simulink library "MCI_lib"  (Simulink 7.5)
settings: Solver=ode45  StartTime=0.0  StopTime=10.0  RelTol=1e-3
values from neighbouring files (symbols this model uses):
  pMCI_bool_MotCtrlTqLimEna_C = Simulink.Parameter    [MCI_par.m]
  pMCI_m_TireDiam_C = Simulink.Parameter    [MCI_par.m]
  pMCI_Nm_DrvTqLim_C = Simulink.Parameter    [MCI_par.m]
  pMCI_Nm_RcpTqLim_C = Simulink.Parameter    [MCI_par.m]
  pMCI_ratio_DrvEff_MAP = Simulink.Parameter    [MCI_par.m]
  pMCI_ratio_KmPerHrToMtrPerSec_C = Simulink.Parameter    [MCI_par.m]
  pMCI_ratio_TrsmRat_C = Simulink.Parameter    [MCI_par.m]
  pMCI_rpm_InsteadVld_C = Simulink.Parameter    [MCI_par.m]
  pMCI_s_NoOfSec_C = Simulink.Parameter    [MCI_par.m]
undefined symbols (not defined in the file or in its folder): MotCtrlWrkStsTyp, p_bool_False_M, p_bool_True_M, p_st_DrvModeFlg_C
libraries: BaseOperationLib_Browser x79, PES_CZ_FAW x6, simulink x1
(part 2 of 2)

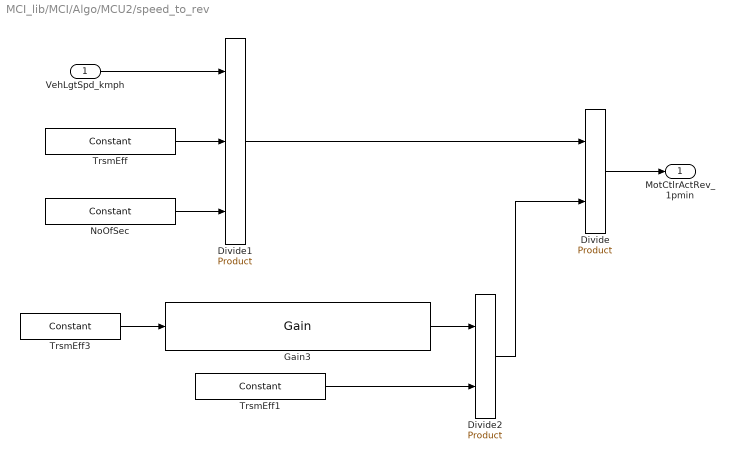
== system MCI_lib/MCI/Algo/MCU2/speed_to_rev ==
  VehLgtSpd_kmph : Inport
  Divide : BaseOperationLib_Browser/Math Operations Changed/Product  Inputs=*/  Multiplication=Element-wise(.*)  OutMin=[]  OutMax=[]  OutDataType=fixdt(1,16,0)  OutScaling=[]
  Divide1 : BaseOperationLib_Browser/Math Operations Changed/Product  Inputs=***  Multiplication=Element-wise(.*)  OutMin=[]  OutMax=[]  OutDataType=fixdt(1,16,0)  OutScaling=[]
  Divide2 : BaseOperationLib_Browser/Math Operations Changed/Product  Inputs=**  Multiplication=Element-wise(.*)  OutMin=[]  OutMax=[]  OutDataType=fixdt(1,16,0)  OutScaling=[]
  Gain3 : BaseOperationLib_Browser/Math Operations Changed/Gain  Gain=pMCI_ratio_KmPerHrToMtrPerSec_C  Multiplication=Element-wise(K.*u)  ParamMin=[]  ParamMax=[]  ParameterDataType=fixdt(1, 16)  ParameterScalingMode=Best Precision: Matrix-wise  ParameterScaling=2^0  OutMin=[]  OutMax=[]  OutDataType=fixdt(1, 16)  OutScaling=2^0
  NoOfSec : BaseOperationLib_Browser/Sources&Sinks/Constant  Value=pMCI_s_NoOfSec_C  OutMin=[]  OutMax=[]  OutDataTypeMode=single  OutDataType=fixdt(1, 16)  ConRadixGroup=Use specified scaling  OutScaling=2^0  OutDataTypeStr=single
  TrsmEff : BaseOperationLib_Browser/Sources&Sinks/Constant  Value=pMCI_ratio_TrsmRat_C  OutMin=[]  OutMax=[]  OutDataTypeMode=single  OutDataType=fixdt(1, 16)  ConRadixGroup=Use specified scaling  OutScaling=2^0  OutDataTypeStr=single
  TrsmEff1 : BaseOperationLib_Browser/Sources&Sinks/Constant  Value=pMCI_m_TireDiam_C  OutMin=[]  OutMax=[]  OutDataTypeMode=single  OutDataType=fixdt(1, 16)  ConRadixGroup=Use specified scaling  OutScaling=2^0  OutDataTypeStr=single
  TrsmEff3 : BaseOperationLib_Browser/Sources&Sinks/Constant  Value=pi  OutMin=[]  OutMax=[]  OutDataTypeMode=single  OutDataType=fixdt(1, 16)  ConRadixGroup=Use specified scaling  OutScaling=2^0  OutDataTypeStr=single
  MotCtlrActRev_1pmin : Outport
  wires:
  TrsmEff1/1 -> Divide2/2
  Divide/1 -> MotCtlrActRev_1pmin/1
  VehLgtSpd_kmph/1 -> Divide1/1
  TrsmEff/1 -> Divide1/2
  NoOfSec/1 -> Divide1/3
  TrsmEff3/1 -> Gain3/1
  Gain3/1 -> Divide2/1
  Divide1/1 -> Divide/1
  Divide2/1 -> Divide/2
